simulink model "InputShape"  (R2020b)
settings: Solver=VariableStepAuto  StartTime=0.0  StopTime=25  RelTol=1e-3
undefined symbols (not defined in the file): sigbuilder_block
settings Model: Creator=32186  LastModifiedBy=32186

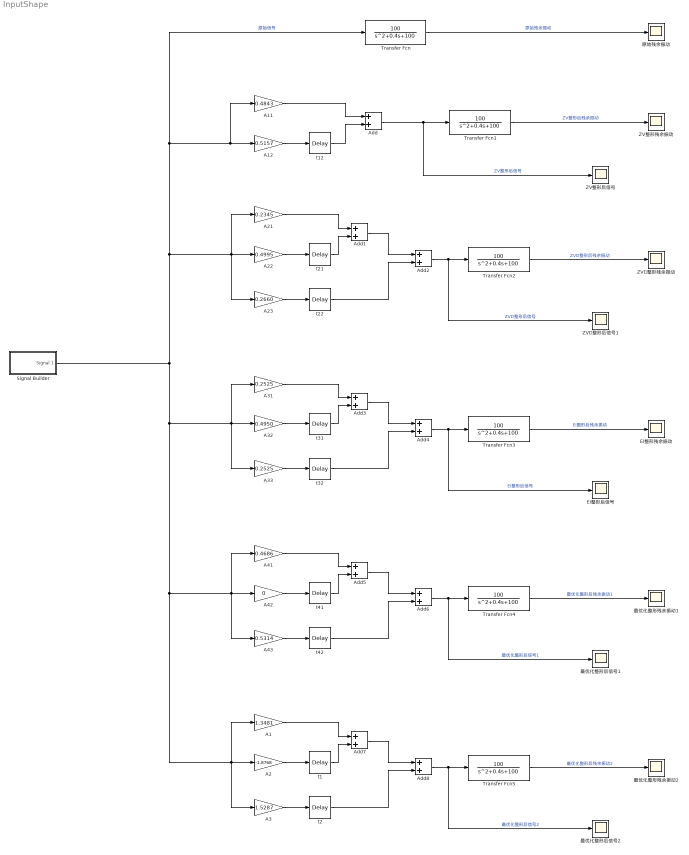
== system InputShape ==
  A1 : Gain  Gain=1.3481
  A11 : Gain  Gain=0.4843
  A12 : Gain  Gain=0.5157
  A2 : Gain  Gain=-1.8768
  A21 : Gain  Gain=0.2345
  A22 : Gain  Gain=0.4995
  A23 : Gain  Gain=0.2660
  A3 : Gain  Gain=1.5287
  A31 : Gain  Gain=0.2525
  A32 : Gain  Gain=0.4950
  A33 : Gain  Gain=0.2525
  A41 : Gain  Gain=0.4686
  A42 : Gain  Gain=0
  A43 : Gain  Gain=0.5314
  Add{,1..8} (9 alike) : Sum
  EI整形后信号 : Scope
  EI整形残余振动 : Scope
  Signal Builder : Subsystem  Tag=STV Subsys  LoadFcn=sigbuilder_block('load');  StartFcn=sigbuilder_block('start');  StopFcn=sigbuilder_block('stop');  ClipboardFcn=sigbuilder_block('clipboard');  mask(Sigbuilder block){tuvar=[0:10]}
      mask help: Simulink:masks:SigbuilderBlock_MD
      mask init:
      | if ~strcmp(get_param(bdroot(gcbh),'SimulationStatus'),'stopped') tuvar = sigbuilder_block('maskInit'); end
      settings: CopyFcn=sigbuilder_block('copy');  DeleteFcn=sigbuilder_block('delete');  ModelCloseFcn=sigbuilder_block('modelClose');  PreSaveFcn=sigbuilder_block('preSave');  PauseFcn=sigbuilder_block('pause');  ContinueFcn=sigbuilder_block('continue');  NameChangeFcn=sigbuilder_block('namechange');  OpenFcn=sigbuilder_block('open',[437.6 199.2 550.4 400 ]);  CloseFcn=sigbuilder_block('close');
      mask Display: plot(0, 0, 100, 100,[2, 2, 32, 32, 2], [68, 8, 8, 68, 68],[32, 2], [38, 38], [32, 19, 2],[53, 60, 44], [32, 17, 17, 2],[16, 16, 31, 31]);txt = getActiveGroup(gcbh);text(2, 100, txt,'verticalAlignment', 'top');
  Transfer Fcn{,1..5} (6 alike) : TransferFcn  Numerator=[100]  Denominator=[1 0.4 100]
  ZVD整形后信号1 : Scope
  ZVD整形残余振动 : Scope
  ZV整形后信号 : Scope
  ZV整形残余振动 : Scope
  t1 : TransportDelay  DelayTime=0.0786
  t{12,21,31,42} (4 alike) : TransportDelay  DelayTime=0.3142
  t2 : TransportDelay  DelayTime=0.1571
  t22 : TransportDelay  DelayTime=0.6284
  t32 : TransportDelay  DelayTime=0.6284
  t41 : TransportDelay  DelayTime=0.1571
  原始残余振动 : Scope
  最优化整形后信号1 : Scope
  最优化整形后信号2 : Scope
  最优化整形残余振动1 : Scope
  最优化整形残余振动2 : Scope
  wires:
  A12/1 -> t12/1
  A11/1 -> Add/1
  t12/1 -> Add/2
  Add/1 -> ZV整形后信号/1, Transfer Fcn1/1  "ZV整形后信号"
  Transfer Fcn1/1 -> ZV整形残余振动/1  "ZV整形后残余振动"
  Transfer Fcn/1 -> 原始残余振动/1  "原始残余振动"
  Transfer Fcn2/1 -> ZVD整形残余振动/1  "ZVD整形后残余振动"
  A21/1 -> Add1/1
  A22/1 -> t21/1
  t21/1 -> Add1/2
  t22/1 -> Add2/2
  A23/1 -> t22/1
  Add1/1 -> Add2/1
  Add2/1 -> ZVD整形后信号1/1, Transfer Fcn2/1  "ZVD整形后信号"
  Add3/1 -> Add4/1
  t32/1 -> Add4/2
  A32/1 -> t31/1
  Add4/1 -> EI整形后信号/1, Transfer Fcn3/1  "EI整形后信号"
  A31/1 -> Add3/1
  Transfer Fcn3/1 -> EI整形残余振动/1  "EI整形后残余振动"
  A33/1 -> t32/1
  t31/1 -> Add3/2
  A41/1 -> Add5/1
  Add6/1 -> 最优化整形后信号1/1, Transfer Fcn4/1  "最优化整形后信号1"
  Transfer Fcn4/1 -> 最优化整形残余振动1/1  "最优化整形后残余振动1"
  A43/1 -> t42/1
  A42/1 -> t41/1
  t41/1 -> Add5/2
  t42/1 -> Add6/2
  Add5/1 -> Add6/1
  Add7/1 -> Add8/1
  t1/1 -> Add7/2
  t2/1 -> Add8/2
  A2/1 -> t1/1
  A3/1 -> t2/1
  A1/1 -> Add7/1
  Signal Builder/1(Signal 1) -> Transfer Fcn/1, A11/1, A12/1, A23/1, A22/1, A21/1, A42/1, A43/1, A41/1, A1/1, A2/1, A3/1, A31/1, A33/1, A32/1  "原始信号"
  Transfer Fcn5/1 -> 最优化整形残余振动2/1  "最优化整形后残余振动2"
  Add8/1 -> 最优化整形后信号2/1, Transfer Fcn5/1  "最优化整形后信号2"

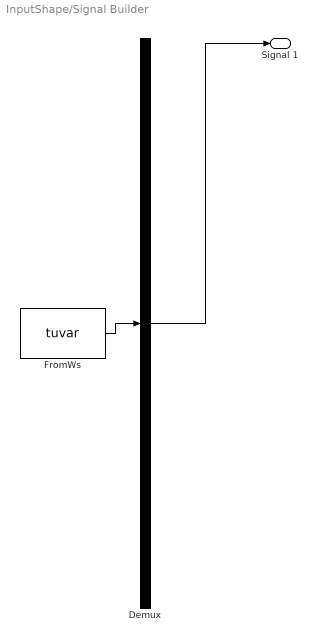
== system InputShape/Signal Builder ==
  Demux : Demux  Tag=STV Demux  Outputs=1
      settings: DisplayOption=none
  FromWs : FromWorkspace  Tag=STV FromWs  VariableName=tuvar
      SigBuilderData=|
      | common.afterFinalStr = 'Extrapolate'
      | common.sampleTime = 0
      | dataSet.timeRange = [0 30]
      | dataSet.name = 'Group 1'
      | sbobj.Groups.Name = 'Group 1'
      | sbobj.Groups.Signals.Name = 'Signal 1'
      | sbobj.Groups.Signals.XData = [0 2 2.2 2.8 3 30]
      | sbobj.Groups.Signals.YData = [0 0 1 1 0 0]
      | sbobj.Groups.TimeRange = [0 30]
  Signal 1 : Outport  Tag=STV Outport
  wires:
  Demux/1 -> Signal 1/1
  FromWs/1 -> Demux/1
